simulink model "FullAssembly1"  (R2024b)
settings: Solver=VariableStepAuto  StartTime=0.0  StopTime=15  RelTol=1e-3
model workspace: external: MATLAB File C:\Users\20221837\Documents\Personal_Projects\Mini_Ranka\Mark1\Simulations\Matlab_Sim_Gravity\FullAssembly_DataFile.m (data not in the file)
undefined symbols (not defined in the file): smiData, X, Y, Z
libraries: sm_lib x48, nesl_utility x12, slpidlib x3
(part 2 of 2)

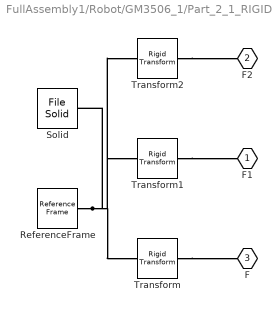
== system FullAssembly1/Robot/GM3506_1/Part_2_1_RIGID ==
  ReferenceFrame : sm_lib/Frames and Transforms/Reference Frame
  Solid : sm_lib/Body Elements/File Solid  ExtGeomFileName=Part 21.step  UnitType=FromFile  ExtGeomFileUnits=m  StepReaderType=HEX  ExportConvexHullGeometry=off  InertiaType=Custom  BasedOnType=DensityFromFile  Density=1000  DensityUnits=kg/m^3  Mass=smiData.Solid(2).mass  MassUnits=g  CenterOfMass=smiData.Solid(2).CoM  CenterOfMassUnits=m  MomentsOfInertia=smiData.Solid(2).MoI  MomentsOfInertiaUnits=g*m^2  ProductsOfInertia=smiData.Solid(2).PoI  ProductsOfInertiaUnits=g*m^2  GraphicType=FromGeometry  MarkerShape=Sphere  MarkerSize=10  GraphicVisPropType=SimpleVisualProperties  GraphicDiffuseColor=smiData.Solid(2).color  GraphicOpacity=smiData.Solid(2).opacity  GraphicSpecularColor=[0.5 0.5 0.5 1.0]  GraphicAmbientColor=[0.15 0.15 0.15 1.0]  GraphicEmissiveColor=[0.0 0.0 0.0 1.0]  GraphicShininess=75  DoExposeReferenceFrame=on  SerializedFrames=<Frames/>
  Transform : sm_lib/Frames and Transforms/Rigid Transform  RotationMethod=ArbitraryAxis  FollAlignAxisA=+X  BaseAlignAxisA=+Y  FollAlignAxisB=+Y  BaseAlignAxisB=+Z  RotationStandardAxis=+Z  RotationAngle=smiData.RigidTransform(1).angle  RotationAngleUnits=rad  RotationArbitraryAxis=smiData.RigidTransform(1).axis  RotationSequenceAxes=FollowerAxes  RotationSequence=XYX  RotationSequenceAngles=[0 0 0]  RotationSequenceAnglesUnits=deg  RotationMatrix=[1 0 0;0 1 0;0 0 1]  Quaternion=[1 0 0 0]  TranslationMethod=Cartesian  TranslationCartesianOffset=smiData.RigidTransform(1).translation  TranslationCartesianOffsetUnits=m  TranslationStandardAxis=+Z  TranslationStandardOffset=0  TranslationStandardOffsetUnits=m  TranslationROffset=0  TranslationROffsetUnits=m  TranslationThetaOffset=0  TranslationThetaOffsetUnits=deg  TranslationZOffset=0  TranslationZOffsetUnits=m
  Transform1 : sm_lib/Frames and Transforms/Rigid Transform  RotationMethod=ArbitraryAxis  FollAlignAxisA=+X  BaseAlignAxisA=+Y  FollAlignAxisB=+Y  BaseAlignAxisB=+Z  RotationStandardAxis=+Z  RotationAngle=smiData.RigidTransform(6).angle  RotationAngleUnits=rad  RotationArbitraryAxis=smiData.RigidTransform(6).axis  RotationSequenceAxes=FollowerAxes  RotationSequence=XYX  RotationSequenceAngles=[0 0 0]  RotationSequenceAnglesUnits=deg  RotationMatrix=[1 0 0;0 1 0;0 0 1]  Quaternion=[1 0 0 0]  TranslationMethod=Cartesian  TranslationCartesianOffset=smiData.RigidTransform(6).translation  TranslationCartesianOffsetUnits=m  TranslationStandardAxis=+Z  TranslationStandardOffset=0  TranslationStandardOffsetUnits=m  TranslationROffset=0  TranslationROffsetUnits=m  TranslationThetaOffset=0  TranslationThetaOffsetUnits=deg  TranslationZOffset=0  TranslationZOffsetUnits=m
  Transform2 : sm_lib/Frames and Transforms/Rigid Transform  RotationMethod=ArbitraryAxis  FollAlignAxisA=+X  BaseAlignAxisA=+Y  FollAlignAxisB=+Y  BaseAlignAxisB=+Z  RotationStandardAxis=+Z  RotationAngle=smiData.RigidTransform(10).angle  RotationAngleUnits=rad  RotationArbitraryAxis=smiData.RigidTransform(10).axis  RotationSequenceAxes=FollowerAxes  RotationSequence=XYX  RotationSequenceAngles=[0 0 0]  RotationSequenceAnglesUnits=deg  RotationMatrix=[1 0 0;0 1 0;0 0 1]  Quaternion=[1 0 0 0]  TranslationMethod=Cartesian  TranslationCartesianOffset=smiData.RigidTransform(10).translation  TranslationCartesianOffsetUnits=m  TranslationStandardAxis=+Z  TranslationStandardOffset=0  TranslationStandardOffsetUnits=m  TranslationROffset=0  TranslationROffsetUnits=m  TranslationThetaOffset=0  TranslationThetaOffsetUnits=deg  TranslationZOffset=0  TranslationZOffsetUnits=m
  F1 : PMIOPort  Side=Left
  F2 : PMIOPort  Port=2  Side=Left
  F : PMIOPort  Port=3  Side=Right
  connections:
  ReferenceFrame/RConn1 -- Solid/RConn1 -- Transform/LConn1 -- Transform1/LConn1 -- Transform2/LConn1
  Transform/RConn1 -- F/RConn1
  Transform1/RConn1 -- F1/RConn1
  Transform2/RConn1 -- F2/RConn1

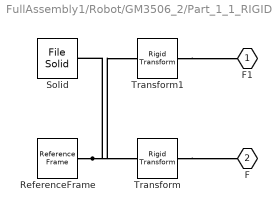
== system FullAssembly1/Robot/GM3506_2/Part_1_1_RIGID ==
  ReferenceFrame : sm_lib/Frames and Transforms/Reference Frame
  Solid : sm_lib/Body Elements/File Solid  ExtGeomFileName=Part 13.step  UnitType=FromFile  ExtGeomFileUnits=m  StepReaderType=HEX  ExportConvexHullGeometry=off  InertiaType=Custom  BasedOnType=DensityFromFile  Density=1000  DensityUnits=kg/m^3  Mass=smiData.Solid(3).mass  MassUnits=g  CenterOfMass=smiData.Solid(3).CoM  CenterOfMassUnits=m  MomentsOfInertia=smiData.Solid(3).MoI  MomentsOfInertiaUnits=g*m^2  ProductsOfInertia=smiData.Solid(3).PoI  ProductsOfInertiaUnits=g*m^2  GraphicType=FromGeometry  MarkerShape=Sphere  MarkerSize=10  GraphicVisPropType=SimpleVisualProperties  GraphicDiffuseColor=smiData.Solid(3).color  GraphicOpacity=smiData.Solid(3).opacity  GraphicSpecularColor=[0.5 0.5 0.5 1.0]  GraphicAmbientColor=[0.15 0.15 0.15 1.0]  GraphicEmissiveColor=[0.0 0.0 0.0 1.0]  GraphicShininess=75  DoExposeReferenceFrame=on  SerializedFrames=<Frames/>
  Transform : sm_lib/Frames and Transforms/Rigid Transform  RotationMethod=ArbitraryAxis  FollAlignAxisA=+X  BaseAlignAxisA=+Y  FollAlignAxisB=+Y  BaseAlignAxisB=+Z  RotationStandardAxis=+Z  RotationAngle=smiData.RigidTransform(2).angle  RotationAngleUnits=rad  RotationArbitraryAxis=smiData.RigidTransform(2).axis  RotationSequenceAxes=FollowerAxes  RotationSequence=XYX  RotationSequenceAngles=[0 0 0]  RotationSequenceAnglesUnits=deg  RotationMatrix=[1 0 0;0 1 0;0 0 1]  Quaternion=[1 0 0 0]  TranslationMethod=Cartesian  TranslationCartesianOffset=smiData.RigidTransform(2).translation  TranslationCartesianOffsetUnits=m  TranslationStandardAxis=+Z  TranslationStandardOffset=0  TranslationStandardOffsetUnits=m  TranslationROffset=0  TranslationROffsetUnits=m  TranslationThetaOffset=0  TranslationThetaOffsetUnits=deg  TranslationZOffset=0  TranslationZOffsetUnits=m
  Transform1 : sm_lib/Frames and Transforms/Rigid Transform  RotationMethod=ArbitraryAxis  FollAlignAxisA=+X  BaseAlignAxisA=+Y  FollAlignAxisB=+Y  BaseAlignAxisB=+Z  RotationStandardAxis=+Z  RotationAngle=smiData.RigidTransform(15).angle  RotationAngleUnits=rad  RotationArbitraryAxis=smiData.RigidTransform(15).axis  RotationSequenceAxes=FollowerAxes  RotationSequence=XYX  RotationSequenceAngles=[0 0 0]  RotationSequenceAnglesUnits=deg  RotationMatrix=[1 0 0;0 1 0;0 0 1]  Quaternion=[1 0 0 0]  TranslationMethod=Cartesian  TranslationCartesianOffset=smiData.RigidTransform(15).translation  TranslationCartesianOffsetUnits=m  TranslationStandardAxis=+Z  TranslationStandardOffset=0  TranslationStandardOffsetUnits=m  TranslationROffset=0  TranslationROffsetUnits=m  TranslationThetaOffset=0  TranslationThetaOffsetUnits=deg  TranslationZOffset=0  TranslationZOffsetUnits=m
  F1 : PMIOPort  Side=Left
  F : PMIOPort  Port=2  Side=Left
  connections:
  ReferenceFrame/RConn1 -- Solid/RConn1 -- Transform/LConn1 -- Transform1/LConn1
  Transform/RConn1 -- F/RConn1
  Transform1/RConn1 -- F1/RConn1

== system FullAssembly1/Robot/GM3506_2/Part_2_1_RIGID ==
  ReferenceFrame : sm_lib/Frames and Transforms/Reference Frame
  Solid : sm_lib/Body Elements/File Solid  ExtGeomFileName=Part 21.step  UnitType=FromFile  ExtGeomFileUnits=m  StepReaderType=HEX  ExportConvexHullGeometry=off  InertiaType=Custom  BasedOnType=DensityFromFile  Density=1000  DensityUnits=kg/m^3  Mass=smiData.Solid(2).mass  MassUnits=g  CenterOfMass=smiData.Solid(2).CoM  CenterOfMassUnits=m  MomentsOfInertia=smiData.Solid(2).MoI  MomentsOfInertiaUnits=g*m^2  ProductsOfInertia=smiData.Solid(2).PoI  ProductsOfInertiaUnits=g*m^2  GraphicType=FromGeometry  MarkerShape=Sphere  MarkerSize=10  GraphicVisPropType=SimpleVisualProperties  GraphicDiffuseColor=smiData.Solid(2).color  GraphicOpacity=smiData.Solid(2).opacity  GraphicSpecularColor=[0.5 0.5 0.5 1.0]  GraphicAmbientColor=[0.15 0.15 0.15 1.0]  GraphicEmissiveColor=[0.0 0.0 0.0 1.0]  GraphicShininess=75  DoExposeReferenceFrame=on  SerializedFrames=<Frames/>
  Transform : sm_lib/Frames and Transforms/Rigid Transform  RotationMethod=ArbitraryAxis  FollAlignAxisA=+X  BaseAlignAxisA=+Y  FollAlignAxisB=+Y  BaseAlignAxisB=+Z  RotationStandardAxis=+Z  RotationAngle=smiData.RigidTransform(1).angle  RotationAngleUnits=rad  RotationArbitraryAxis=smiData.RigidTransform(1).axis  RotationSequenceAxes=FollowerAxes  RotationSequence=XYX  RotationSequenceAngles=[0 0 0]  RotationSequenceAnglesUnits=deg  RotationMatrix=[1 0 0;0 1 0;0 0 1]  Quaternion=[1 0 0 0]  TranslationMethod=Cartesian  TranslationCartesianOffset=smiData.RigidTransform(1).translation  TranslationCartesianOffsetUnits=m  TranslationStandardAxis=+Z  TranslationStandardOffset=0  TranslationStandardOffsetUnits=m  TranslationROffset=0  TranslationROffsetUnits=m  TranslationThetaOffset=0  TranslationThetaOffsetUnits=deg  TranslationZOffset=0  TranslationZOffsetUnits=m
  Transform1 : sm_lib/Frames and Transforms/Rigid Transform  RotationMethod=ArbitraryAxis  FollAlignAxisA=+X  BaseAlignAxisA=+Y  FollAlignAxisB=+Y  BaseAlignAxisB=+Z  RotationStandardAxis=+Z  RotationAngle=smiData.RigidTransform(13).angle  RotationAngleUnits=rad  RotationArbitraryAxis=smiData.RigidTransform(13).axis  RotationSequenceAxes=FollowerAxes  RotationSequence=XYX  RotationSequenceAngles=[0 0 0]  RotationSequenceAnglesUnits=deg  RotationMatrix=[1 0 0;0 1 0;0 0 1]  Quaternion=[1 0 0 0]  TranslationMethod=Cartesian  TranslationCartesianOffset=smiData.RigidTransform(13).translation  TranslationCartesianOffsetUnits=m  TranslationStandardAxis=+Z  TranslationStandardOffset=0  TranslationStandardOffsetUnits=m  TranslationROffset=0  TranslationROffsetUnits=m  TranslationThetaOffset=0  TranslationThetaOffsetUnits=deg  TranslationZOffset=0  TranslationZOffsetUnits=m
  F1 : PMIOPort  Side=Left
  F : PMIOPort  Port=2  Side=Right
  connections:
  ReferenceFrame/RConn1 -- Transform/LConn1 -- Transform1/LConn1 -- Solid/RConn1
  Transform/RConn1 -- F/RConn1
  Transform1/RConn1 -- F1/RConn1

== matlab function FullAssembly1/Forward Kinematics ==
function [xc, yc, zc] = fcn(theta1, theta2, theta3)
l1=0.0488;
l2=0.20;
l3=0.20;
xc = -sin(theta1)*(l2*cos(theta2)+l3*cos(theta2-theta3));
yc = cos(theta1)*(l2*cos(theta2)+l3*cos(theta2-theta3));
zc = l1-l2*sin(theta2)-l3*sin(theta2-theta3);

== matlab function FullAssembly1/Trajectory ==
function [th1, th2, th3, thd, thdd]  = fcn(T, th1des, th2des, th3des, t)
if (t<=T)
% Define the given times and boundary conditions
t0 = 0; % Initial time
tf = T; % Final time

qth10 = 0; % Initial position
qth20 = 0;
qth30 = 0;
v0 = 0; % Initial velocity
a0 = 0; % Initial acceleration
th1f = th1des; % Final position
th2f = th2des;
th3f = th3des;
vf = 0; % Final velocity
af = 0; % Final acceleration

A = [1  t0   t0^2    t0^3    t0^4    t0^5;
     0  1    2*t0    3*t0^2  4*t0^3  5*t0^4;
     0  0    2       6*t0    12*t0^2 20*t0^3;
     1  tf   tf^2    tf^3    tf^4    tf^5;
     0  1    2*tf    3*tf^2  4*tf^3  5*tf^4;
     0  0    2       6*tf    12*tf^2 20*tf^3];
bth1 = [qth10; v0; a0; th1f; vf; af];
coefficientsth1 = A \ bth1;

ax0 = coefficientsth1(1);
ax1 = coefficientsth1(2);
ax2 = coefficientsth1(3);
ax3 = coefficientsth1(4);
ax4 = coefficientsth1(5);
ax5 = coefficientsth1(6);
th1=ax0+ax1*t+ax2*t^2+ax3*t^3+ax4*t^4+ax5*t^5;
th1d=ax1+2*ax2*t+3*ax3*t^2+4*ax4*t^3+5*ax5*t^4;
th1dd=2*ax2+6*ax3*t+12*ax4*t^2+20*ax5*t^3;

bth2 = [qth20; v0; a0; th2f; vf; af];
coefficientsth2 = A \ bth2;

ay0 = coefficientsth2(1);
ay1 = coefficientsth2(2);
ay2 = coefficientsth2(3);
ay3 = coefficientsth2(4);
ay4 = coefficientsth2(5);
ay5 = coefficientsth2(6);
th2=ay0+ay1*t+ay2*t^2+ay3*t^3+ay4*t^4+ay5*t^5;
th2d=ay1+2*ay2*t+3*ay3*t^2+4*ay4*t^3+5*ay5*t^4;
th2dd=2*ay2+6*ay3*t+12*ay4*t^2+20*ay5*t^3;

bth3 = [qth30; v0; a0; th3f; vf; af];
coefficientsth3 = A \ bth3;

az0 = coefficientsth3(1);
az1 = coefficientsth3(2);
az2 = coefficientsth3(3);
az3 = coefficientsth3(4);
az4 = coefficientsth3(5);
az5 = coefficientsth3(6);
th3=az0+az1*t+az2*t^2+az3*t^3+az4*t^4+az5*t^5;
th3d=az1+2*az2*t+3*az3*t^2+4*az4*t^3+5*az5*t^4;
th3dd=2*az2+6*az3*t+12*az4*t^2+20*az5*t^3;
thd=[th1d; th2d; th3d];
thdd=[th1dd; th2dd; th3dd];
else
th1=th1des;
th2=th2des;
th3=th3des;
thd=[0;0;0];
thdd=[0; 0; 0];
end

== matlab function FullAssembly1/Inverse Kinematics ==
function [theta1, theta2, theta3] = fcn(x, y, z)

% IK
l1=0.0488;
l2=0.20;
l3=0.20;
r=sqrt(x^2+y^2);
theta1 = atan2(x,y)-pi/2;
theta3 = atan2(-sqrt(1-((r^2+(-z+l1)^2 -l2^2 -l3^2)/ (2*l2*l3))^2), (r^2+(-z+l1)^2 -l2^2 -l3^2)/ (2*l2*l3));
theta2 = atan2(-z+l1, r) + atan2(l3*sin(theta3), l2 + l3*cos(theta3));

== matlab function FullAssembly1/Gravity FF ==
function g = fcn(th1, th2, th3)

g = -[ 0;
        (0.27152609*cos(th2) + 0.04188947*cos(th2-th3));
        -0.04188947*cos(th2-th3)];

== matlab function FullAssembly1/Inertia FF ==
function D = fcn(th1, th2, th3)
D11 = 0.002467*cos(2.0*th2) ...
    - 0.00002835*sin(2.0*th2) ...
    + 0.0008537*cos(th3) ...
    + 0.0008537*cos(2.0*th2 - 1.0*th3) ...
    + 0.0002465*cos(2.0*th2 - 2.0*th3) ...
    - 0.00002180*sin(2.0*th2 - 2.0*th3) ...
    + 0.002837;

% row 1, col 2 (symmetric with row 2, col 1)
D12 = 3.325e-05 * sin(th2 - 1.0*th3) ...
     + 3.543e-07 * cos(th2) ...
     + 7.980e-05 * sin(th2);

% row 1, col 3 (and row 3, col 1)
D13 = -3.325e-05 * sin(th2 - 1.0*th3);

% row 2, col 2
D22 = 0.001707 * cos(th3) ...
    + 0.005447;

% row 2, col 3 (and row 3, col 2)
D23 = -0.0008537 * cos(th3) ...
      - 0.0005012;

% row 3, col 3
D33 = 0.0005012;

% assemble symmetric matrix
D = [ D11,  D12,  D13;
      D12,  D22,  D23;
      D13,  D23,  D33 ];

== matlab function FullAssembly1/Coriolis FF ==
function C = fcn(th1, th2, th3, thd1, thd2, thd3)

% 3x3 Coriolis matrix C (numeric coefficients rounded to 4 significant digits)
C = [
    thd3*(2.180e-05*cos(2.*th2 - 2.*th3) - 4.268e-04*sin(th3) + 4.268e-04*sin(2.*th2 - th3) + 2.465e-04*sin(2.*th2 - 2.*th3)) ...
  - thd2*(2.835e-05*cos(2.*th2) + 2.467e-03*sin(2.*th2) + 2.180e-05*cos(2.*th2 - 2.*th3) + 8.537e-04*sin(2.*th2 - th3) + 2.465e-04*sin(2.*th2 - 2.*th3)), ...
    thd2*(3.325e-05*cos(th2 - th3) + 7.980e-05*cos(th2) - 3.544e-07*sin(th2)) ...
  - 3.325e-05*thd3*cos(th2 - th3) ...
  - thd1*(2.835e-05*cos(2.*th2) + 2.467e-03*sin(2.*th2) + 2.180e-05*cos(2.*th2 - 2.*th3) + 8.537e-04*sin(2.*th2 - th3) + 2.465e-04*sin(2.*th2 - 2.*th3)), ...
    3.325e-05*thd3*cos(th2 - th3) - 3.325e-05*thd2*cos(th2 - th3) ...
  + thd1*(2.180e-05*cos(2.*th2 - 2.*th3) - 4.268e-04*sin(th3) + 4.268e-04*sin(2.*th2 - th3) + 2.465e-04*sin(2.*th2 - 2.*th3))
;
    thd1*(2.835e-05*cos(2.*th2) + 2.467e-03*sin(2.*th2) + 2.180e-05*cos(2.*th2 - 2.*th3) + 8.537e-04*sin(2.*th2 - th3) + 2.465e-04*sin(2.*th2 - 2.*th3)), ...
   -8.537e-04*thd3*sin(th3), ...
    8.537e-04*thd3*sin(th3) - 8.537e-04*thd2*sin(th3)
;
  - thd1*(2.180e-05*cos(2.*th2 - 2.*th3) - 4.268e-04*sin(th3) + 4.268e-04*sin(2.*th2 - th3) + 2.465e-04*sin(2.*th2 - 2.*th3)), ...
    8.537e-04*thd2*sin(th3), ...
    0
];
